simulink model "Openloop_dashboard"  (R2020b)
settings: Solver=FixedStepAuto  StartTime=0.0  StopTime=Inf  RelTol=1e-3  EnableMultiTasking=on
undefined symbols (not defined in the file or in its folder): serial
libraries: instrumentlib x2
settings Model: SimulationMode=accelerator  ExtModeTrigDuration=8  Creator=Mladen  LastModifiedBy=hites
settings SolverCC: AutoInsertRateTranBlk=on
settings DataIOCC: ReturnWorkspaceOutputs=off
settings OptimizationCC: DefaultUnderspecifiedDataType=single  EnhancedBackFolding=on  PassReuseOutputArgsAs=Individual arguments  MaxStackSize=512  OptimizeBlockOrder=speed  DifferentSizesBufferReuse=on  OptimizationCustomize=off  EfficientTunableParamExpr=on
settings DebuggingCC: ParameterTunabilityLossMsg=error  ArithmeticOperatorsInVariantConditions=warning
settings HardwareCC: ProdBitPerChar=16  ProdBitPerInt=16  ProdBitPerPointer=32  ProdBitPerSizeT=32  ProdBitPerPtrDiffT=32  ProdLargestAtomicInteger=Integer  ProdLargestAtomicFloat=None  ProdWordSize=16  ProdLongLongMode=on  ProdHWDeviceType=Texas Instruments->C2000
settings SFSimCC: MATLABDynamicMemAlloc=off  CustomCodeUndefinedFunction=UseInterfaceOnly
settings RTWCC: Description=Embedded Coder  SystemTargetFile=ert.tlc  HardwareBoard=TI Piccolo F28027/F28027F LaunchPad  TemplateMakefile=ert_default_tmf  GenerateReport=on  Toolchain=Texas Instruments Code Composer Studio (C2000)  IncludeHyperlinkInReport=on  LaunchReport=on  GenerateTraceInfo=on  GenerateTraceReport=on  GenerateTraceReportSl=on  GenerateTraceReportSf=on  GenerateTraceReportEml=on
settings CodeAppCC: ForceParamTrailComments=on  IgnoreCustomStorageClasses=off  OperatorAnnotations=on  SimulinkDataObjDesc=on  SFDataObjDesc=on  InsertBlockDesc=on
settings ERTTargetCC: CodeReplacementLibrary=TI C28x

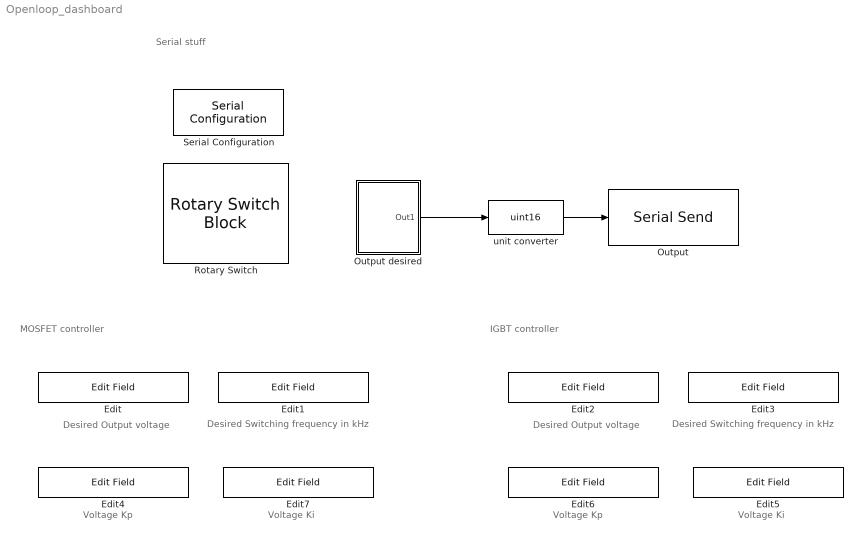
== system Openloop_dashboard ==
  note: Desired Switching frequency in kHz
  note: Desired Output voltage
  note: Serial stuff
  note: MOSFET controller
  note: Desired Output voltage
  note: IGBT controller
  note: Desired Switching frequency in kHz
  note: Voltage Kp
  note: Voltage Ki
  note: Voltage Kp
  note: Voltage Ki
  Edit{,1..7} (8 alike) : EditField  LabelPosition=Hide  ShowInitialText=on  Alignment=Center
  Output : instrumentlib/Serial Send  ComPortMenu=<Please select a port...>  ComPort=COM3  ObjConstructor=serial('COM3');  Header=S  Terminator=E  EnableBlockingMode=on
  Output desired : Subsystem
  Rotary Switch : RotarySwitchBlock
      settings: Values={{'OFF', 'IGBT', 'MOSFET'}, [0 1 2]}
  Serial Configuration : instrumentlib/Serial Configuration  Priority=-200000  ComPortMenu=<Please select a port...>  ComPort=COM3  ObjConstructor=serial('COM3');  BaudRate=9600  DataBits=8  Parity=none  StopBits=1  FlowControl=hardware  Timeout=2  ByteOrder=LittleEndian
  unit converter : DataTypeConversion  OutDataTypeStr=uint16  ConvertRealWorld=Stored Integer (SI)
  wires:
  unit converter/1 -> Output/1
  Output desired/1(Out1) -> unit converter/1

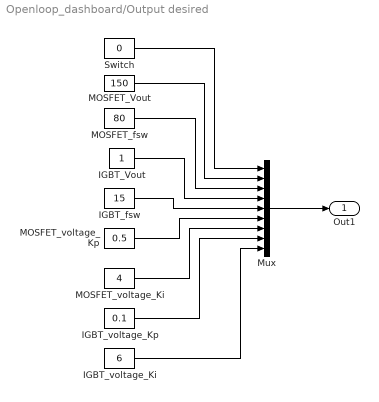
== system Openloop_dashboard/Output desired ==
  IGBT_Vout : Constant
  IGBT_fsw : Constant  Value=15
  IGBT_voltage_Ki : Constant  Value=6
  IGBT_voltage_Kp : Constant  Value=0.1
  MOSFET_Vout : Constant  Value=150
  MOSFET_fsw : Constant  Value=80
  MOSFET_voltage_Ki : Constant  Value=4
  MOSFET_voltage_Kp : Constant  Value=0.5
  Mux : Mux  Inputs=9
  Switch : Constant  Value=0
  Out1 : Outport
  wires:
  IGBT_Vout/1 -> Mux/4
  IGBT_fsw/1 -> Mux/5
  Mux/1 -> Out1/1
  MOSFET_Vout/1 -> Mux/2
  Switch/1 -> Mux/1
  MOSFET_fsw/1 -> Mux/3
  MOSFET_voltage_Kp/1 -> Mux/6
  MOSFET_voltage_Ki/1 -> Mux/7
  IGBT_voltage_Kp/1 -> Mux/8
  IGBT_voltage_Ki/1 -> Mux/9
